simulink model "RECTIFIER"  (R2024a)
settings: Solver=VariableStepAuto  StartTime=0.0  StopTime=0.08  RelTol=1e-3
libraries: spsDiodeLib x6, spsVoltageMeasurementLib x6, spsACVoltageSourceLib x3, spsCurrentMeasurementLib x1, spsSeriesRLCBranchLib x1, sps_lib x1
settings Model: Creator=ianyl  LastModifiedBy=ianyl

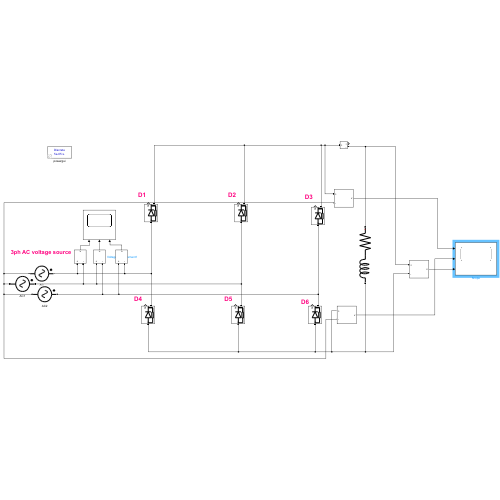
[thumbnail: Simulink's stored preview of the top-level diagram]
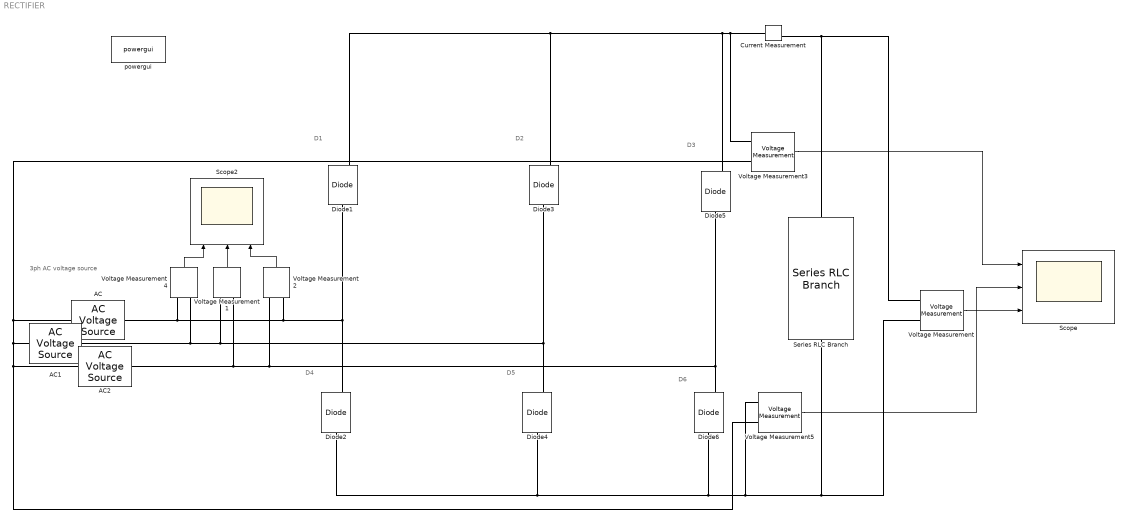
== system RECTIFIER ==
  note: D4
  note: 3ph AC voltage source
  note: D1
  note: D5
  note: D2
  note: D6
  note: D3
  AC : spsACVoltageSourceLib/AC Voltage Source  Amplitude=220  Phase=0  Frequency=50  SampleTime=0  Measurements=None  BusType=swing  Pref=10e3  Qref=0  Qmin=-inf  Qmax=+inf
  AC1 : spsACVoltageSourceLib/AC Voltage Source  Amplitude=220  Phase=-120  Frequency=50  SampleTime=0  Measurements=None  BusType=swing  Pref=10e3  Qref=0  Qmin=-inf  Qmax=+inf
  AC2 : spsACVoltageSourceLib/AC Voltage Source  Amplitude=220  Phase=-240  Frequency=50  SampleTime=0  Measurements=None  BusType=swing  Pref=10e3  Qref=0  Qmin=-inf  Qmax=+inf
  Current Measurement : spsCurrentMeasurementLib/Current Measurement  PhasorSimulation=off  OutputType=Complex  PSBequivalent=0
  Diode{1..6} (6 alike) : spsDiodeLib/Diode  Ron=0.001  Lon=0  Vf=0.8  IC=0  UseSnubber=0  Rs=500  Cs=250e-9  Measurements=on
  Scope : Scope  NumInputPorts=3
  Scope2 : Scope  NumInputPorts=3
  Series RLC Branch : spsSeriesRLCBranchLib/Series RLC Branch  LConnTagsString=__new0  RConnTagsString=__new0  BranchType=RL  Resistance=50  Inductance=0.9  SetiL0=off  InitialCurrent=0  Capacitance=1e-6  Setx0=off  InitialVoltage=0  Measurements=None
  Voltage Measurement{,1..5} (6 alike) : spsVoltageMeasurementLib/Voltage Measurement  PhasorSimulation=off  OutputType=Complex  PSBequivalent=0
  powergui : sps_lib/powergui  Priority=1  SimulationMode=Discrete  SampleTime=50e-6  frequency=60  Iterations=50  frequencyindice=50  Pbase=100e6  ErrMax=1e-4  UnitsV=kV  UnitsW=MW  buscounter=0  FunctionMessages=off  echomessages=off  EnableUseOfTLC=off  CurrentSourceSwitches=off  DisableSnubberDevices=off  DisableRonSwitches=off  DisableVfSwitches=off  DisplayEquations=off  AutomaticDiscreteSolvers=off  SolverType=Tustin/Backward Euler (TBE)  Interpol=off  ExternalGateDelay=off  methode=off  Ts=100  x0status=blocks  SPID=on  SwTol=0  HookPort=off  NonlinearTolerance=1e-4  nMaxIteration=100  ContinueOnMaxIteration=off  RestoreLinks=warning  ResistiveCurrentMeasurement=off  Frange=[0:2:500]  Ylog=off  Xlog=on  ShowGrid=off  save=off  variable=ZData  structure=0  ZoomFFT=off  StartTime=0.0  cycles=1  DisplayStyle=1  fundamental=60  FreqAxis=off  MaxFrequency=1000  frequencyindicesteady=1  RmsSteady=1  display=off
  wires:
  Voltage Measurement4/1 -> Scope2/1
  Voltage Measurement/1 -> Scope/3
  Voltage Measurement1/1 -> Scope2/2
  Voltage Measurement2/1 -> Scope2/3
  Voltage Measurement3/1 -> Scope/1
  Voltage Measurement5/1 -> Scope/2
  connections:
  Current Measurement/LConn1 -- Voltage Measurement3/LConn1 -- Diode5/RConn1 -- Diode3/RConn1 -- Diode1/RConn1
  Voltage Measurement/LConn1 -- Series RLC Branch/LConn1 -- Current Measurement/RConn1
  Diode1/LConn1 -- Voltage Measurement2/LConn2 -- AC/RConn1 -- Voltage Measurement4/LConn1 -- Diode2/RConn1
  Voltage Measurement/LConn2 -- Series RLC Branch/RConn1 -- Diode4/LConn1 -- Diode2/LConn1 -- Diode6/LConn1 -- Voltage Measurement5/LConn1
  Diode4/RConn1 -- Diode3/LConn1 -- Voltage Measurement4/LConn2 -- AC1/RConn1 -- Voltage Measurement1/LConn1
  Diode6/RConn1 -- Voltage Measurement2/LConn1 -- AC2/RConn1 -- Voltage Measurement1/LConn2 -- Diode5/LConn1
  AC2/LConn1 -- Voltage Measurement5/LConn2 -- AC/LConn1 -- Voltage Measurement3/LConn2 -- AC1/LConn1
